simulink model "house_with_onoff_sim"  (R2020b)
settings: Solver=ode45  StartTime=0.0  StopTime=4*3600  RelTol=1e-3  EnableMultiTasking=on
undefined symbols (not defined in the file): C_R, H, K, Q_F_ON, Q_H, t_a, t_init, t_R_set, tau_F, tau_s
libraries: simulink_extras x1
settings Model: Creator=sgt  LastModifiedBy=Hammer
settings DataIOCC: LimitDataPoints=on  SaveFormat=Array  SignalLoggingSaveFormat=ModelDataLogs
settings OptimizationCC: ExpressionDepthLimit=2147483647  InitFltsAndDblsToZero=on  LifeSpan=inf
settings DebuggingCC: SaveWithParameterizedLinksMsg=none  UnderspecifiedInitializationDetection=Classic  MergeDetectMultiDrivingBlocksExec=none  SignalResolutionControl=TryResolveAllWithWarning  SolverPrmCheckMsg=warning  MultiTaskDSMMsg=warning  MultiTaskCondExecSysMsg=none  StateNameClashWarn=warning  SFUnexpectedBacktrackingDiag=warning  SFNoUnconditionalDefaultTransitionDiag=warning  SFExecutionAtInitializationDiag=none  ArithmeticOperatorsInVariantConditions=warning
settings HardwareCC: ProdBitPerPointer=32  ProdBitPerSizeT=32  ProdBitPerPtrDiffT=32  ProdLargestAtomicFloat=None  ProdIntDivRoundTo=Undefined  ProdEndianess=Unspecified  ProdWordSize=32  ProdHWDeviceType=32-bit Generic
settings ModelReferenceCC: PropagateSignalLabelsOutOfModel=off
settings SFSimCC: SimUseLocalCustomCode=off  CustomCodeUndefinedFunction=UseInterfaceOnly
settings RTWCC: RTWUseLocalCustomCode=off
settings CodeAppCC: StateflowObjectComments=on
settings GRTTargetCC: TargetFcnLib=ansi_tfl_tmw.mat  TargetLangStandard=C89/C90 (ANSI)  CombineOutputUpdateFcns=off  GRTInterface=on
settings ConfigComp: CovMetricSettings=dw  CovSaveCumulativeToWorkspaceVar=on  CovSaveSingleToWorkspaceVar=on  CovExternalEMLEnable=off

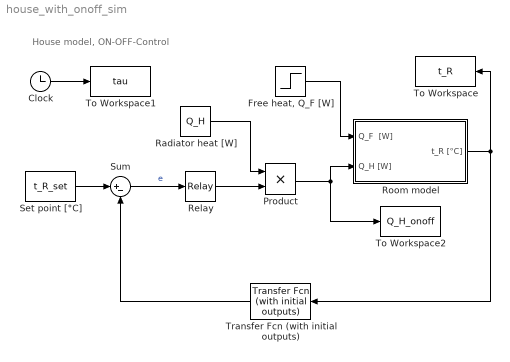
== system house_with_onoff_sim ==
  note: House model, ON-OFF-Control
  Clock : Clock
  "Free heat, Q_F [W]" : Step  Time=tau_F  After=Q_F_ON  SampleTime=0
  Product : Product  RndMeth=Zero
  Radiator heat [W] : Constant  Value=Q_H
  Relay : Relay  OnSwitchValue=H/2  OffSwitchValue=-H/2
  Room model : Subsystem
  Set point [°C] : Constant  Value=t_R_set
  Sum : Sum  Inputs=|+-
  To Workspace : ToWorkspace  VariableName=t_R  SampleTime=-1
  To Workspace1 : ToWorkspace  VariableName=tau  SampleTime=-1
  To Workspace2 : ToWorkspace  VariableName=Q_H_onoff  SampleTime=-1
  Transfer Fcn (with initial outputs) : simulink_extras/Additional Linear/Transfer Fcn (with initial outputs)  N=[1]  D="[tau_s  1]"  Y0=t_init  U0=0
  wires:
  Clock/1 -> To Workspace1/1
  "Free heat, Q_F [W]"/1 -> Room model/1(Q_F  [W])
  Room model/1(t_R [°C]) -> To Workspace/1, Transfer Fcn (with initial outputs)/1
  Product/1 -> Room model/2(Q_H [W]), To Workspace2/1
  Relay/1 -> Product/2
  Radiator heat [W]/1 -> Product/1
  Set point [°C]/1 -> Sum/1
  Transfer Fcn (with initial outputs)/1 -> Sum/2
  Sum/1 -> Relay/1  "e"

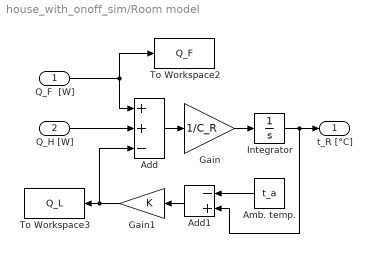
== system house_with_onoff_sim/Room model ==
  Q_F  [W] : Inport
  Q_H [W] : Inport  Port=2
  Add : Sum  Inputs=++-
  Add1 : Sum  Inputs=-+
  Amb. temp. : Constant  Value=t_a
  Gain : Gain  Gain=1/C_R
  Gain1 : Gain  Gain=K
  Integrator : Integrator  InitialCondition=t_init
  To Workspace2 : ToWorkspace  VariableName=Q_F  SampleTime=-1
  To Workspace3 : ToWorkspace  VariableName=Q_L  SampleTime=-1
  t_R [°C] : Outport
  wires:
  Integrator/1 -> Add1/2, t_R [°C]/1
  Gain/1 -> Integrator/1
  Add/1 -> Gain/1
  Q_F  [W]/1 -> To Workspace2/1, Add/1
  Amb. temp./1 -> Add1/1
  Add1/1 -> Gain1/1
  Gain1/1 -> Add/3, To Workspace3/1
  Q_H [W]/1 -> Add/2
